simulink model "mbd3_02"  (R2020b)
settings: Solver=VariableStepAuto  StartTime=0.0  StopTime=10.0  RelTol=1e-3
settings Model: Creator=karth  LastModifiedBy=karth

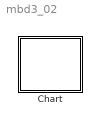
== system mbd3_02 ==
  Chart : Stateflow chart  TreatAsAtomicUnit=on

== stateflow chart mbd3_02/Chart ==
  note: [coin==1]{soda=0}
  state git_0
  state got_nickel
  note: [coin==2]{soda=1}
  note: [coin==1]{soda=1}
  note: [coin==1]{soda=1}
  note: [coin==2]{soda=1}
  note: [coin==1]{soda=0}
  state got_dime
  (default) -> git_0
  git_0 -> got_nickel [order 1]
  got_nickel -> git_0 [order 2]
  got_dime -> git_0 [order 2]
  git_0 -> got_dime [order 2]
  got_nickel -> got_dime [order 1]
  got_dime -> got_nickel [order 1]
